simulink model "Esempio8_s"  (R2021b)
settings: Solver=VariableStepAuto  StartTime=0.0  StopTime=10.0  RelTol=1e-3
undefined symbols (not defined in the file): A, B, C, K, x0
settings Model: Creator=Steph  LastModifiedBy=Steph

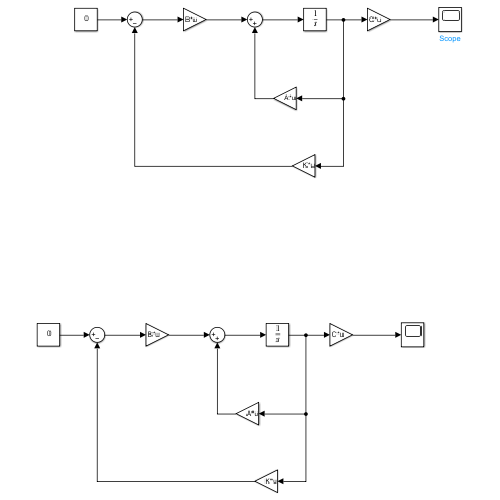
[thumbnail: Simulink's stored preview of the top-level diagram]
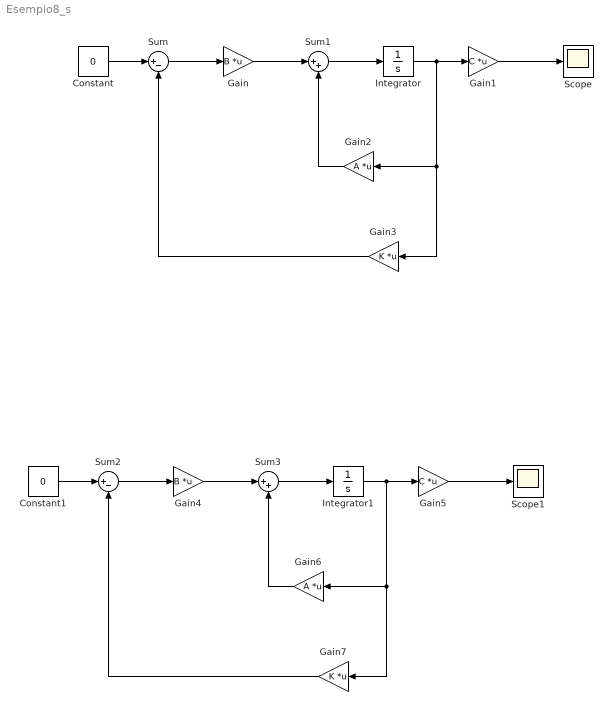
== system Esempio8_s ==
  Constant : Constant  Value=0
  Constant1 : Constant  Value=0
  Gain : Gain  Gain=B  Multiplication=Matrix(K*u)
  Gain1 : Gain  Gain=C  Multiplication=Matrix(K*u)
  Gain2 : Gain  Gain=A  Multiplication=Matrix(K*u)
  Gain3 : Gain  Gain=K  Multiplication=Matrix(K*u)
  Gain4 : Gain  Gain=B  Multiplication=Matrix(K*u)
  Gain5 : Gain  Gain=C  Multiplication=Matrix(K*u)
  Gain6 : Gain  Gain=A  Multiplication=Matrix(K*u)
  Gain7 : Gain  Gain=K  Multiplication=Matrix(K*u)
  Integrator : Integrator  InitialCondition=x0
  Integrator1 : Integrator  InitialCondition=[0.4; 0; 0.8; 0]
  Scope : Scope
  Scope1 : Scope
  Sum : Sum  Inputs=|+-
  Sum1 : Sum  Inputs=|++
  Sum2 : Sum  Inputs=|+-
  Sum3 : Sum  Inputs=|++
  wires:
  Integrator/1 -> Gain3/1, Gain2/1, Gain1/1
  Gain1/1 -> Scope/1
  Gain2/1 -> Sum1/2
  Gain3/1 -> Sum/2
  Sum/1 -> Gain/1
  Gain/1 -> Sum1/1
  Constant/1 -> Sum/1
  Sum1/1 -> Integrator/1
  Gain4/1 -> Sum3/1
  Sum2/1 -> Gain4/1
  Sum3/1 -> Integrator1/1
  Gain6/1 -> Sum3/2
  Integrator1/1 -> Gain7/1, Gain6/1, Gain5/1
  Constant1/1 -> Sum2/1
  Gain7/1 -> Sum2/2
  Gain5/1 -> Scope1/1
